simulink model "Raschet_G"  (Simulink 7.7)
settings: Solver=ode3  StartTime=0.0  StopTime=1  FixedStep=0.1  RelTol=1e-3
settings Model: Creator=Natalia  LastModifiedBy=Natalia

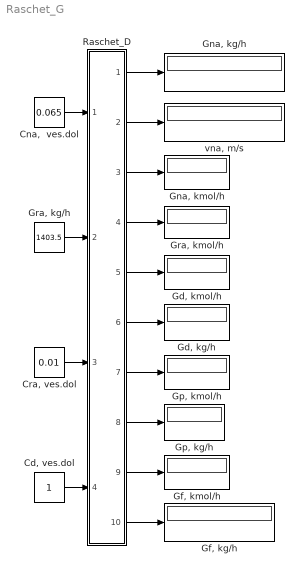
== system Raschet_G ==
  "Cd, ves.dol" : Constant
  "Cna,  ves.dol" : Constant  Value=0.065
  "Cra, ves.dol" : Constant  Value=0.01
  "Gd, kg/h" : Display
  "Gd, kmol/h" : Display
  "Gf, kg/h" : Display
  "Gf, kmol/h" : Display
  "Gna, kg/h" : Display
  "Gna, kmol/h" : Display
  "Gp, kg/h" : Display
  "Gp, kmol/h" : Display
  "Gra, kg/h" : Constant  Value=1403.5
  "Gra, kmol/h" : Display
  Raschet_D : Subsystem
  "vna, m/s" : Display
  wires:
  "Cna,  ves.dol"/1 -> Raschet_D/1(In1)
  "Cra, ves.dol"/1 -> Raschet_D/3(In3)
  "Cd, ves.dol"/1 -> Raschet_D/4(In4)
  "Gra, kg/h"/1 -> Raschet_D/2(In2)
  Raschet_D/6(Out6) -> "Gd, kg/h"/1
  Raschet_D/8(Out8) -> "Gp, kg/h"/1
  Raschet_D/10(Out10) -> "Gf, kg/h"/1
  Raschet_D/2(Out2) -> "vna, m/s"/1
  Raschet_D/1(Out1) -> "Gna, kg/h"/1
  Raschet_D/3(Out3) -> "Gna, kmol/h"/1
  Raschet_D/4(Out4) -> "Gra, kmol/h"/1
  Raschet_D/5(Out5) -> "Gd, kmol/h"/1
  Raschet_D/7(Out7) -> "Gp, kmol/h"/1
  Raschet_D/9(Out9) -> "Gf, kmol/h"/1

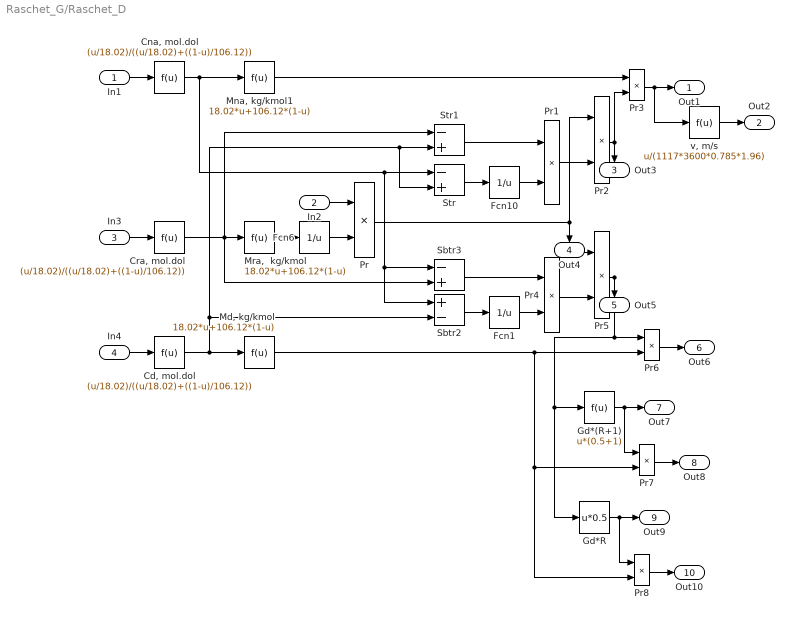
== system Raschet_G/Raschet_D ==
  In1 : Inport
  In2 : Inport  Port=2
  In3 : Inport  Port=3
  In4 : Inport  Port=4
  "Cd, mol.dol" : Fcn  Expr=(u/18.02)/((u/18.02)+((1-u)/106.12))
  "Cna, mol.dol" : Fcn  Expr=(u/18.02)/((u/18.02)+((1-u)/106.12))
  "Cra, mol.dol" : Fcn  Expr=(u/18.02)/((u/18.02)+((1-u)/106.12))
  Fcn1 : Fcn  Expr=1/u
  Fcn10 : Fcn  Expr=1/u
  Fcn6 : Fcn  Expr=1/u
  Gd*(R+1) : Fcn  Expr=u*(0.5+1)
  Gd*R : Fcn  Expr=u*0.5
  "Md, kg/kmol" : Fcn  Expr=18.02*u+106.12*(1-u)
  "Mna, kg/kmol1" : Fcn  Expr=18.02*u+106.12*(1-u)
  "Mra,  kg/kmol" : Fcn  Expr=18.02*u+106.12*(1-u)
  Pr{,1..8} (9 alike) : Product  RndMeth=Zero
  Sbtr2 : Sum  Inputs=+-
  Sbtr3 : Sum  Inputs=-+
  Str : Sum  Inputs=-+
  Str1 : Sum  Inputs=-+
  "v, m/s" : Fcn  Expr=u/(1117*3600*0.785*1.96)
  Out1 : Outport
  Out2 : Outport  Port=2
  Out3 : Outport  Port=3
  Out4 : Outport  Port=4
  Out5 : Outport  Port=5
  Out6 : Outport  Port=6
  Out7 : Outport  Port=7
  Out8 : Outport  Port=8
  Out9 : Outport  Port=9
  Out10 : Outport  Port=10
  wires:
  Pr3/1 -> "v, m/s"/1, Out1/1
  Gd*R/1 -> Pr8/1, Out9/1
  Gd*(R+1)/1 -> Pr7/1, Out7/1
  Sbtr3/1 -> Pr4/1
  Sbtr2/1 -> Fcn1/1
  "Md, kg/kmol"/1 -> Pr6/2, Pr7/2, Pr8/2
  Pr4/1 -> Pr5/2
  Pr5/1 -> Pr6/1, Gd*(R+1)/1, Gd*R/1, Out5/1
  Fcn1/1 -> Pr4/2
  Str1/1 -> Pr1/1
  Pr1/1 -> Pr2/2
  Pr2/1 -> Pr3/2, Out3/1
  Fcn10/1 -> Pr1/2
  Str/1 -> Fcn10/1
  Pr/1 -> Pr2/1, Out4/1, Pr5/1
  Fcn6/1 -> Pr/2
  "Mra,  kg/kmol"/1 -> Fcn6/1
  "Cd, mol.dol"/1 -> "Md, kg/kmol"/1, Str1/2, Str/2, Sbtr2/2
  "Cra, mol.dol"/1 -> "Mra,  kg/kmol"/1, Str1/1, Sbtr3/2
  "Cna, mol.dol"/1 -> "Mna, kg/kmol1"/1, Str/1, Sbtr3/1, Sbtr2/1
  "Mna, kg/kmol1"/1 -> Pr3/1
  In1/1 -> "Cna, mol.dol"/1
  "v, m/s"/1 -> Out2/1
  In2/1 -> Pr/1
  In3/1 -> "Cra, mol.dol"/1
  Pr6/1 -> Out6/1
  In4/1 -> "Cd, mol.dol"/1
  Pr7/1 -> Out8/1
  Pr8/1 -> Out10/1
